simulink model "kinematic_model_control"  (R2014a)
settings: Solver=ode45  StartTime=0.0  StopTime=100  FixedStep=0.01  RelTol=1e-3
values from neighbouring files (symbols this model uses):
  K = 5*diag(ones(1,3))    [init.m]
  l2 = 0.40    (= 0.4)    [init.m]    (also in jacobian_numeric.m = 0.2; singularity_plot.m = 0.2; testing_IGM.m = 0.2; trajectory_generation.m = 0.2)
  l3 = 0.20    (= 0.2)    [init.m]    (also in jacobian_numeric.m = 0.15; singularity_plot.m = 0.15; testing_IGM.m = 0.4; trajectory_generation.m = 0.15)
settings Model: Creator=subodh  LastModifiedBy=subodh
settings DebuggingCC: MergeDetectMultiDrivingBlocksExec=error  FrameProcessingCompatibilityMsg=error

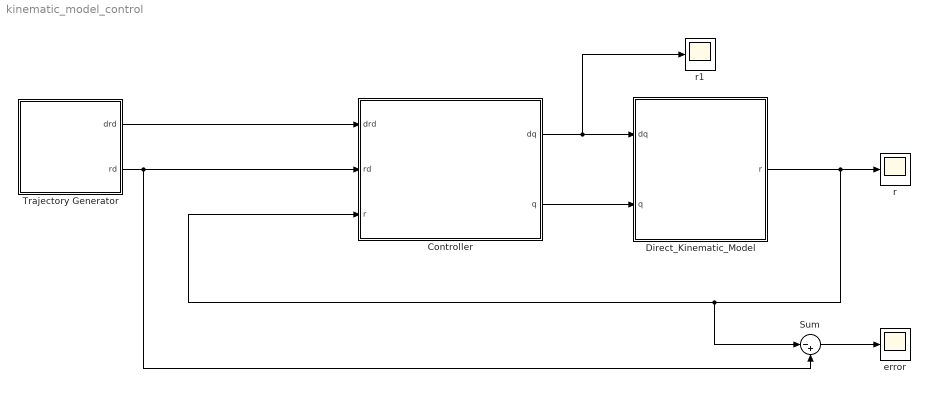
== system kinematic_model_control ==
  Controller : Subsystem
  Direct_Kinematic_Model : Subsystem
  Sum : Sum  Inputs=|-+
  Trajectory Generator : Subsystem
  error : Scope
      settings: YMin=1.38778e-17  YMax=0.225
  r : Scope
      settings: YMin=1.38778e-17  YMax=0.225
  r1 : Scope
      settings: YMin=1.38778e-17  YMax=0.225  SaveName=ScopeData2
  wires:
  Controller/1(dq) -> r1/1, Direct_Kinematic_Model/1(dq)
  Controller/2(q) -> Direct_Kinematic_Model/2(q)
  Direct_Kinematic_Model/1(r) -> r/1, Controller/3(r), Sum/1
  Trajectory Generator/1(drd) -> Controller/1(drd)
  Trajectory Generator/2(rd) -> Controller/2(rd), Sum/2
  Sum/1 -> error/1

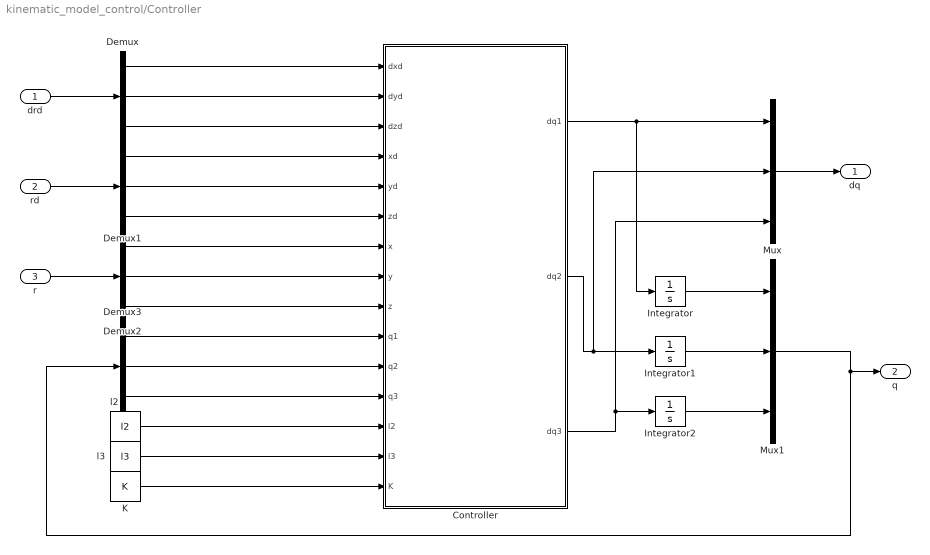
== system kinematic_model_control/Controller ==
  drd : Inport
  rd : Inport  Port=2
  r : Inport  Port=3
  Controller : MATLAB Function  TreatAsAtomicUnit=on
  Demux{,1..3} (4 alike) : Demux  Outputs=3
  Integrator : Integrator  InitialCondition=1.5708
  Integrator1 : Integrator  InitialCondition=0.2987
  Integrator2 : Integrator  InitialCondition=0.7227
  K : Constant  Value=K
  Mux : Mux  Inputs=3
  Mux1 : Mux  Inputs=3
  l2 : Constant  Value=l2
  l3 : Constant  Value=l3
  dq : Outport
  q : Outport  Port=2
  wires:
  Demux/2 -> Controller/2(dyd)
  Demux1/2 -> Controller/5(yd)
  Demux1/1 -> Controller/4(xd)
  Demux3/1 -> Controller/10(q1)
  Demux3/2 -> Controller/11(q2)
  Demux/3 -> Controller/3(dzd)
  Demux2/3 -> Controller/9(z)
  Demux/1 -> Controller/1(dxd)
  Demux1/3 -> Controller/6(zd)
  Demux3/3 -> Controller/12(q3)
  Demux2/2 -> Controller/8(y)
  Demux2/1 -> Controller/7(x)
  drd/1 -> Demux/1
  rd/1 -> Demux1/1
  r/1 -> Demux2/1
  Mux/1 -> dq/1
  Controller/1(dq1) -> Mux/1, Integrator/1
  Controller/2(dq2) -> Mux/2, Integrator1/1
  Controller/3(dq3) -> Mux/3, Integrator2/1
  Integrator/1 -> Mux1/1
  Integrator1/1 -> Mux1/2
  Integrator2/1 -> Mux1/3
  Mux1/1 -> q/1, Demux3/1
  l2/1 -> Controller/13(l2)
  l3/1 -> Controller/14(l3)
  K/1 -> Controller/15(K)

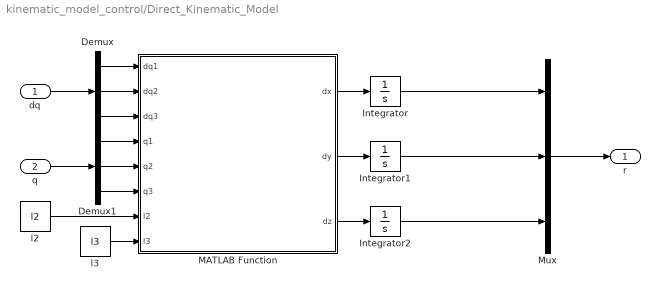
== system kinematic_model_control/Direct_Kinematic_Model ==
  dq : Inport
  q : Inport  Port=2
  Demux : Demux  Outputs=3
  Demux1 : Demux  Outputs=3
  Integrator : Integrator  InitialCondition=0.4
  Integrator1 : Integrator  InitialCondition=0.4
  Integrator2 : Integrator
  MATLAB Function : MATLAB Function  TreatAsAtomicUnit=on
  Mux : Mux  Inputs=3
  l2 : Constant  Value=l2
  l3 : Constant  Value=l3
  r : Outport
  wires:
  MATLAB Function/1(dx) -> Integrator/1
  MATLAB Function/2(dy) -> Integrator1/1
  MATLAB Function/3(dz) -> Integrator2/1
  Integrator1/1 -> Mux/2
  Demux1/1 -> MATLAB Function/4(q1)
  Demux1/2 -> MATLAB Function/5(q2)
  Demux1/3 -> MATLAB Function/6(q3)
  Mux/1 -> r/1
  Demux/1 -> MATLAB Function/1(dq1)
  Demux/2 -> MATLAB Function/2(dq2)
  Demux/3 -> MATLAB Function/3(dq3)
  dq/1 -> Demux/1
  q/1 -> Demux1/1
  Integrator/1 -> Mux/1
  Integrator2/1 -> Mux/3
  l3/1 -> MATLAB Function/8(l3)
  l2/1 -> MATLAB Function/7(l2)

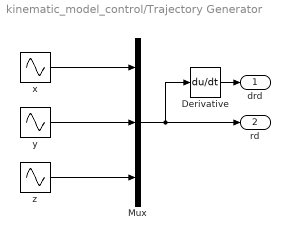
== system kinematic_model_control/Trajectory Generator ==
  Derivative : Derivative
  Mux : Mux  Inputs=3
  x : Sin  Amplitude=0.4  SampleTime=0
  y : Sin  Amplitude=0.4  Phase=22/14  SampleTime=0
  z : Sin  Amplitude=0  Phase=22/14  SampleTime=0
  drd : Outport
  rd : Outport  Port=2
  wires:
  Mux/1 -> rd/1, Derivative/1
  x/1 -> Mux/1
  z/1 -> Mux/3
  Derivative/1 -> drd/1
  y/1 -> Mux/2

== matlab function kinematic_model_control/Controller/Controller ==
  data: dxd input; dyd input; dzd input; xd input; yd input; zd input; x input; y input; z input; q1 input; q2 input; q3 input; dq1 output; dq2 output; dq3 output; l2 input; l3 input; K input
function [dq1, dq2, dq3] = fcn(dxd, dyd, dzd, xd, yd, zd, x, y, z, q1, q2, q3, l2, l3, K)
%#codegen

J = [ 0,            l3*cos(q2 + q3) + l2*cos(q2),          l3*cos(q2 + q3);
  cos(q1)*(l3*cos(q2 + q3) + l2*cos(q2)), -sin(q1)*(l3*sin(q2 + q3) + l2*sin(q2)), -l3*sin(q2 + q3)*sin(q1);
  sin(q1)*(l3*cos(q2 + q3) + l2*cos(q2)),  cos(q1)*(l3*sin(q2 + q3) + l2*sin(q2)),  l3*sin(q2 + q3)*cos(q1)];
Jinv = pinv(J);

dq = Jinv*([dxd; dyd; dzd] + K*([xd; yd; zd] - [x; y; z]));
dq1 = dq(1);
dq2 = dq(2);
dq3 = dq(3);
end

== matlab function kinematic_model_control/Direct_Kinematic_Model/MATLAB Function ==
  data: dq1 input; dq2 input; dq3 input; q1 input; dx output; q2 input; q3 input; dy output; dz output; l2 input; l3 input
function [dx,dy,dz] = fcn(dq1,dq2,dq3, q1, q2, q3, l2, l3)
%#codegen


dr =[ 0,            l3*cos(q2 + q3) + l2*cos(q2),          l3*cos(q2 + q3);
  cos(q1)*(l3*cos(q2 + q3) + l2*cos(q2)), -sin(q1)*(l3*sin(q2 + q3) + l2*sin(q2)), -l3*sin(q2 + q3)*sin(q1);
  sin(q1)*(l3*cos(q2 + q3) + l2*cos(q2)),  cos(q1)*(l3*sin(q2 + q3) + l2*sin(q2)),  l3*sin(q2 + q3)*cos(q1)]...
     *[dq1; dq2; dq3];

dx = dr(1);
dy = dr(2);
dz = dr(3);

end
